simulink model "MappingSimulator"  (R2016a)
settings: Solver=ode3  StartTime=0.0  StopTime=inf  FixedStep=0.2  RelTol=1e-3
values from neighbouring files (symbols this model uses):
  REFMAP = [0 0 0 0 0 0 0 0 0 0 0 0 ... (65536 elements, 256x256)]    [Frontier256.mat]    (also in ParameterSet.m = MAP)
undefined symbols (not defined in the file or in its folder): Data, Data_SL_Info, Header, Info
libraries: robotlib x6, realtime_pacer_lib x1
settings Model: Creator=einar  LastModifiedBy=einar
settings DataIOCC: LimitDataPoints=on
settings OptimizationCC: OptimizeModelRefInitCode=on  LifeSpan=Inf  MaxStackSize=64
settings DebuggingCC: AllowSymbolicDim=off
settings HardwareCC: ProdBitPerPointer=32  ProdLargestAtomicFloat=None  ProdIntDivRoundTo=Undefined  ProdEndianess=Unspecified  ProdWordSize=32  ProdHWDeviceType=Generic->Unspecified (assume 32-bit Generic)
settings ModelReferenceCC: PropagateSignalLabelsOutOfModel=off
settings RTWCC: SystemTargetFile=ert.tlc  HardwareBoard=Robot Operating System (ROS)  TemplateMakefile=ert_default_tmf  Toolchain=Catkin  TargetLang=C++
settings CodeAppCC: IgnoreCustomStorageClasses=off
settings ERTTargetCC: SupportVariableSizeSignals=on  ConvertIfToSwitch=off  SuppressUnreachableDefaultCases=off

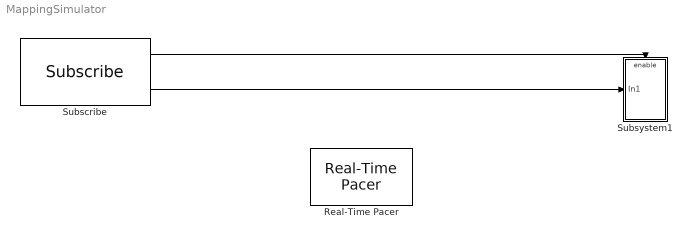
== system MappingSimulator ==
  Real-Time Pacer : realtime_pacer_lib/Real-Time Pacer  simTimePerRealTime=1
  Subscribe : robotlib/Subscribe  SourceLibraryInfo=This block requires Robotics System Toolbox  topicSource=Select from ROS network  topic=/map  messageType=nav_msgs/OccupancyGrid  sampleTime=-1  messageQueueLength=1
  Subsystem1 : Subsystem
  wires:
  Subscribe/2 -> Subsystem1/1(In1)
  Subscribe/1 -> Subsystem1/Enable

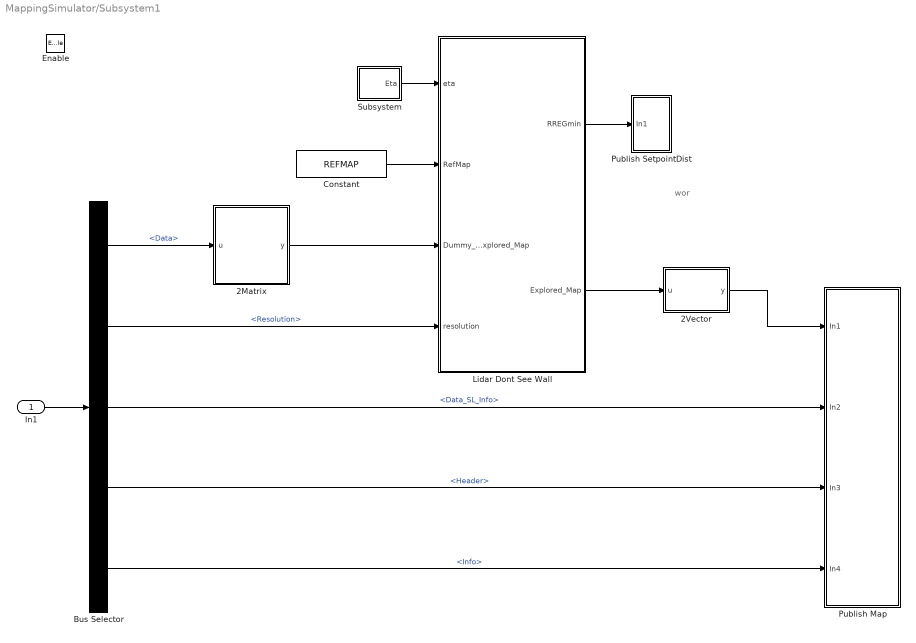
== system MappingSimulator/Subsystem1 ==
  note: wor
  In1 : Inport
  Enable : EnablePort
  2Matrix : MATLAB Function  TreatAsAtomicUnit=on
  2Vector : MATLAB Function  TreatAsAtomicUnit=on
  Bus Selector : BusSelector  OutputSignals=Data,Info.Resolution,Data_SL_Info,Header,Info
  Constant : Constant  Value=REFMAP
  Lidar Dont See Wall : MATLAB Function  TreatAsAtomicUnit=on
  Publish Map : Subsystem
  Publish SetpointDist : Subsystem
  Subsystem : Subsystem
  wires:
  Subsystem/1(Eta) -> Lidar Dont See Wall/1(eta)
  Constant/1 -> Lidar Dont See Wall/2(RefMap)
  Bus Selector/1 -> 2Matrix/1(u)  "<Data>"
  In1/1 -> Bus Selector/1
  Bus Selector/2 -> Lidar Dont See Wall/4(resolution)  "<Resolution>"
  2Matrix/1(y) -> Lidar Dont See Wall/3(Dummy_Explored_Map)
  Lidar Dont See Wall/2(Explored_Map) -> 2Vector/1(u)
  Lidar Dont See Wall/1(RREGmin) -> Publish SetpointDist/1(In1)
  2Vector/1(y) -> Publish Map/1(In1)
  Bus Selector/3 -> Publish Map/2(In2)  "<Data_SL_Info>"
  Bus Selector/4 -> Publish Map/3(In3)  "<Header>"
  Bus Selector/5 -> Publish Map/4(In4)  "<Info>"

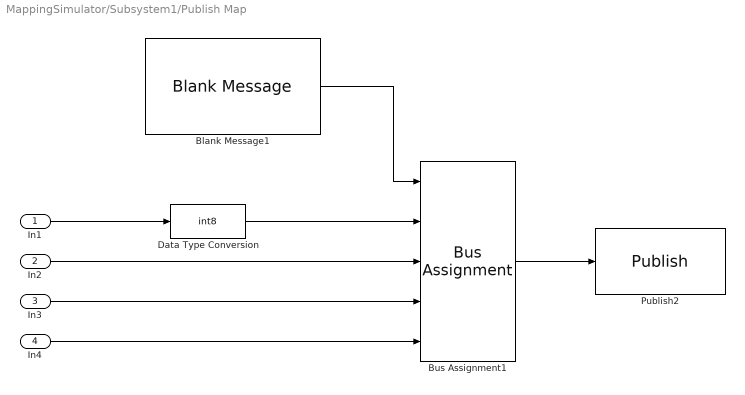
== system MappingSimulator/Subsystem1/Publish Map ==
  In1 : Inport
  In2 : Inport  Port=2
  In3 : Inport  Port=3
  In4 : Inport  Port=4
  Blank Message1 : robotlib/Blank Message  SourceLibraryInfo=This block requires Robotics System Toolbox  messageType=nav_msgs/OccupancyGrid  SampleTime=inf
  Bus Assignment1 : BusAssignment  AssignedSignals=Data,Data_SL_Info,Header,Info
  Data Type Conversion : DataTypeConversion  OutDataTypeStr=int8
  Publish2 : robotlib/Publish  SourceLibraryInfo=This block requires Robotics System Toolbox  topicSource=Specify your own  topic=/map  messageType=nav_msgs/OccupancyGrid  messageQueueLength=1
  wires:
  Bus Assignment1/1 -> Publish2/1
  In2/1 -> Bus Assignment1/3
  Data Type Conversion/1 -> Bus Assignment1/2
  In1/1 -> Data Type Conversion/1
  In4/1 -> Bus Assignment1/5
  Blank Message1/1 -> Bus Assignment1/1
  In3/1 -> Bus Assignment1/4

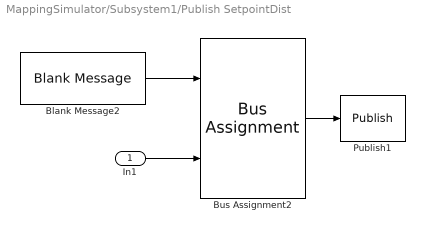
== system MappingSimulator/Subsystem1/Publish SetpointDist ==
  In1 : Inport
  Blank Message2 : robotlib/Blank Message  SourceLibraryInfo=This block requires Robotics System Toolbox  messageType=std_msgs/Float64  SampleTime=inf
  Bus Assignment2 : BusAssignment  AssignedSignals=Data
  Publish1 : robotlib/Publish  SourceLibraryInfo=This block requires Robotics System Toolbox  topicSource=Specify your own  topic=/SetPointDist  messageType=std_msgs/Float64  messageQueueLength=1
  wires:
  Blank Message2/1 -> Bus Assignment2/1
  Bus Assignment2/1 -> Publish1/1
  In1/1 -> Bus Assignment2/2

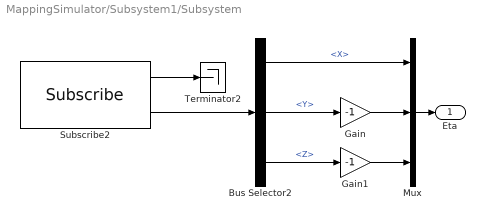
== system MappingSimulator/Subsystem1/Subsystem ==
  Bus Selector2 : BusSelector  OutputSignals=X,Y,Z
  Gain : Gain  Gain=-1
  Gain1 : Gain  Gain=-1
  Mux : Mux  Inputs=3
  Subscribe2 : robotlib/Subscribe  SourceLibraryInfo=This block requires Robotics System Toolbox  topicSource=Specify your own  topic=/Position  messageType=geometry_msgs/Vector3  sampleTime=-1  messageQueueLength=1
  Terminator2 : Terminator
  Eta : Outport
  wires:
  Bus Selector2/1 -> Mux/1  "<X>"
  Subscribe2/2 -> Bus Selector2/1
  Mux/1 -> Eta/1
  Subscribe2/1 -> Terminator2/1
  Bus Selector2/2 -> Gain/1  "<Y>"
  Gain/1 -> Mux/2
  Bus Selector2/3 -> Gain1/1  "<Z>"
  Gain1/1 -> Mux/3

== matlab function MappingSimulator/Subsystem1/2Matrix ==
  data: u input; y output
function y  = fcn(u)
%Transforming occupancy grid from vector to matrix
K=sqrt(size(u,1));
%length(u)^0.5;
MAP=zeros(K,K);
for i=1:K;
    MAP(i,1:K)=u((i-1)*K+1:i*K);
end
y = (MAP);

== matlab function MappingSimulator/Subsystem1/Lidar Dont See Wall ==
  data: RREGmin output; eta input; Explored_Map output; RefMap input; Dummy_Explored_Map input; resolution input
function [RREGmin,Explored_Map] = UpdateUserMap3(eta, RefMap, Dummy_Explored_Map, resolution)
% Updating Explored-map and finding minimal distance to hinders. 
[Height Width]=size(Dummy_Explored_Map);

MID=Height*resolution/2;
RobotPositionY=round((eta(1)+MID)/resolution);
RobotPositionX=round((eta(2)+MID)/resolution);
%%
RREG=zeros(361,1);
MAP=RefMap;

%% Lidar emulator
for Degangle=0:1:360
    Radangle=Degangle*pi/180;
for r=0:1:6.5/resolution;
    XPOS=(RobotPositionX+round(r*cos(Radangle)));
    YPOS=RobotPositionY+round(r*sin(Radangle));
    if ( (XPOS>0) && (XPOS<1+size(Dummy_Explored_Map,2)) && (YPOS>0) &&(YPOS<1+size(Dummy_Explored_Map,1)) )
 
        if MAP(XPOS,YPOS)==2
            Dummy_Explored_Map(XPOS,YPOS)=100;
            rEnd=r;
            for r=0:0.5:rEnd-1;
                XPOS=(RobotPositionX+round(r*cos(Radangle)));
                YPOS=RobotPositionY+round(r*sin(Radangle));
                %if (MAP(XPOS,YPOS)==0 || MAP(XPOS,YPOS)==3)
                if MAP(XPOS,YPOS)==0
                    Dummy_Explored_Map(XPOS,YPOS)=0;
                    if Dummy_Explored_Map(XPOS,YPOS)==-1
                        Dummy_Explored_Map(XPOS,YPOS)=0;
                        %disp('Dummy explored map = -1 ')
                    end 
                end
            end
            RREG(Degangle+1)=double(r*resolution);
            break
        end
    end

end
end
%%

Explored_Map=Dummy_Explored_Map;
if isempty(RREG(RREG~=0))
    RREGmin = 0;
else
    RREGmin=max([0 min(RREG(RREG~=0))]);
end
end

== matlab function MappingSimulator/Subsystem1/2Vector ==
  data: u input; y output
function y = fcn(u)
%Transforming occupancy grid from matrix to vector
L=length(u);
y=zeros(L^2,1);
for i=1:L
y((i-1)*L+1:i*L)=u(i,:);
end

end
